simulink model "ex1"  (R2020a)
settings: Solver=VariableStepAuto  StartTime=0.0  StopTime=10.0  RelTol=1e-3

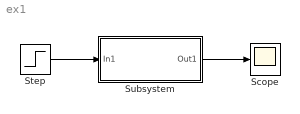
== system ex1 ==
  Scope : Scope
  Step : Step  SampleTime=0
  Subsystem : Subsystem  mask{wn=12, zita=0.5}
      mask prompts: wn "wn="; zita "zita="
      mask Callback wn:
      | if str2num(get_param(gcb,'wn'))<0
      |     error('Introduceti o valoare pozitiva pentru pulsatia naturala')
      | end
      mask Callback zita:
      | if str2num(get_param(gcb,'zita'))<0
      |     error('Introduceti o valoare pozitiva pentru factorul de amortizare')
      | end
  wires:
  Step/1 -> Subsystem/1(In1)
  Subsystem/1(Out1) -> Scope/1

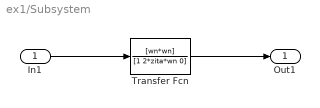
== system ex1/Subsystem ==
  In1 : Inport
  Transfer Fcn : TransferFcn  Numerator=[wn*wn]  Denominator=[1 2*zita*wn 0]
  Out1 : Outport
  wires:
  In1/1 -> Transfer Fcn/1
  Transfer Fcn/1 -> Out1/1
